simulink model "sml_model"  (R2022a)
settings: Solver=VariableStepAuto  StartTime=0.0  StopTime=250  RelTol=1e-3
settings Model: Creator=Huawei  LastModifiedBy=Huawei

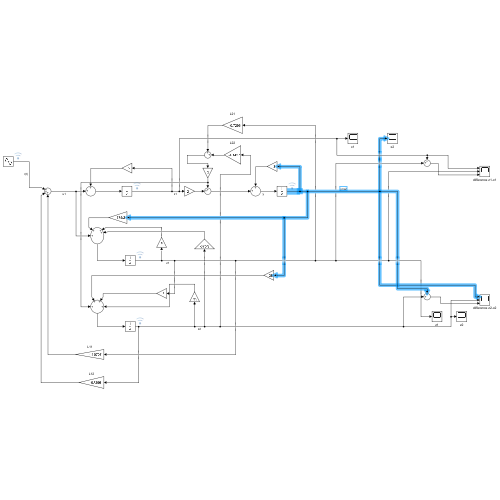
[thumbnail: Simulink's stored preview of the top-level diagram]
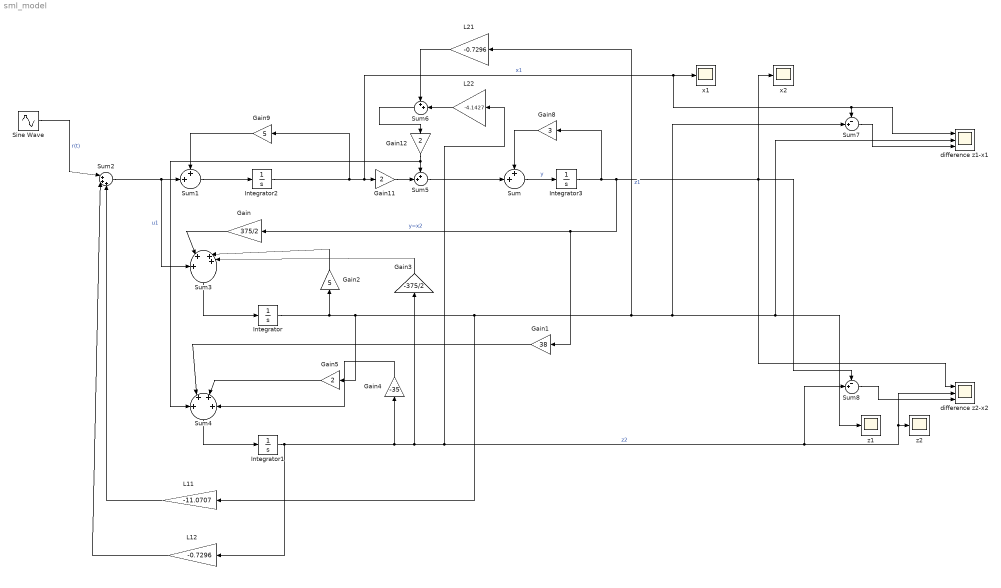
== system sml_model ==
  Gain : Gain  Gain=375/2
  Gain1 : Gain  Gain=38
  Gain11 : Gain  Gain=2
  Gain12 : Gain  Gain=2
  Gain2 : Gain  Gain=5
  Gain3 : Gain  Gain=-375/2
  Gain4 : Gain  Gain=-35
  Gain5 : Gain  Gain=2
  Gain8 : Gain  Gain=3
  Gain9 : Gain  Gain=5
  Integrator : Integrator  InitialCondition=10
  Integrator1 : Integrator  InitialCondition=19
  Integrator2 : Integrator  InitialCondition=-30  ZeroCross=off
  Integrator3 : Integrator  InitialCondition=25  ZeroCross=off
  L11 : Gain  Gain=-11.0707
  L12 : Gain  Gain=-0.7296
  L21 : Gain  Gain=-0.7296
  L22 : Gain  Gain=-4.1427
  Sine Wave : Sin  Amplitude=10  SampleTime=0
  Sum{,1,5..6} (4 alike) : Sum  Inputs=++|
  Sum2 : Sum  Inputs=|+++
  Sum3 : Sum  Inputs=+|+||++|
  Sum4 : Sum  Inputs=+|+|+|+
  Sum7 : Sum  Inputs=-+|
  Sum8 : Sum  Inputs=-+|
  difference z1-x1 : Scope  NumInputPorts=3
  difference z2-x2 : Scope  NumInputPorts=3
  x1 : Scope
  x2 : Scope
  z1 : Scope
  z2 : Scope
  wires:
  Sum8/1 -> difference z2-x2/3
  Sum6/1 -> Gain12/1
  Sum7/1 -> difference z1-x1/3
  Integrator/1 -> Gain5/1, L11/1, z1/1, difference z1-x1/2, Sum7/2, L21/1, Gain2/1  "z1"
  Sum3/1 -> Integrator/1
  Gain12/1 -> Sum5/1, Sum4/1
  Sine Wave/1 -> Sum2/1  "r(t)"
  Integrator3/1 -> Sum8/1, difference z2-x2/1, x2/1, Gain1/1, Gain/1, Gain8/1  "y=x2"
  Integrator1/1 -> difference z2-x2/2, z2/1, Sum8/2, L22/1, Gain3/1, Gain4/1, L12/1  "z2"
  Integrator2/1 -> Gain9/1, x1/1, Sum7/1, difference z1-x1/1, Gain11/1  "x1"
  Gain3/1 -> Sum3/4
  Sum5/1 -> Sum/2
  Gain11/1 -> Sum5/2
  Sum/1 -> Integrator3/1  "y"
  Gain4/1 -> Sum4/4
  Gain2/1 -> Sum3/3
  Sum4/1 -> Integrator1/1
  Sum1/1 -> Integrator2/1
  L12/1 -> Sum2/2
  Gain8/1 -> Sum/1
  Gain/1 -> Sum3/2
  Gain9/1 -> Sum1/1
  Sum2/1 -> Sum3/1, Sum1/2  "u1"
  Gain5/1 -> Sum4/3
  L11/1 -> Sum2/3
  Gain1/1 -> Sum4/2
  L21/1 -> Sum6/1
  L22/1 -> Sum6/2
